simulink library "ammclib_bam_s32k14x"  (Simulink 9.0)
settings: Solver=ode45  StartTime=0.0  StopTime=10.0  RelTol=1e-3
undefined symbols (not defined in the file): f16A1, f16A2, f16B0, f16B1, f16B2, f16C1, f16CC1, f16CC1sc, f16CC1sc_D, f16CC1sc_Q, f16CC1scD, f16CC1scQ, f16CC2, f16CC2sc, f16CC2sc_D, f16CC2sc_Q, f16CC2scD, f16CC2scQ, f16DerivGain, f16EGain, f16FiltCoef, f16HystOff, f16HystOn, f16IGain, f16IntegGain, f16IntegGainFW, f16IntegGainQ, f16Kd, f16Kq, f16Limit, f16LowerLim, f16LowerLimit_D, f16LowerLimit_Q, f16ModIndex, f16OutValOff, f16OutValOn, f16PropGain, f16PropGainFW, f16PropGainQ, f16RampDown, f16RampUp, f16UGain, f16UpperLim, f16UpperLimit, f16UpperLimit_D, f16UpperLimit_Q, f16WIGain, f32A1, f32A2, f32B0, f32B1, f32B2, f32C1, f32CC1, f32CC1sc, f32CC1sc_D, f32CC1sc_Q, f32CC1scD, f32CC1scQ, f32CC2 ... (+122)
(part 2 of 11)

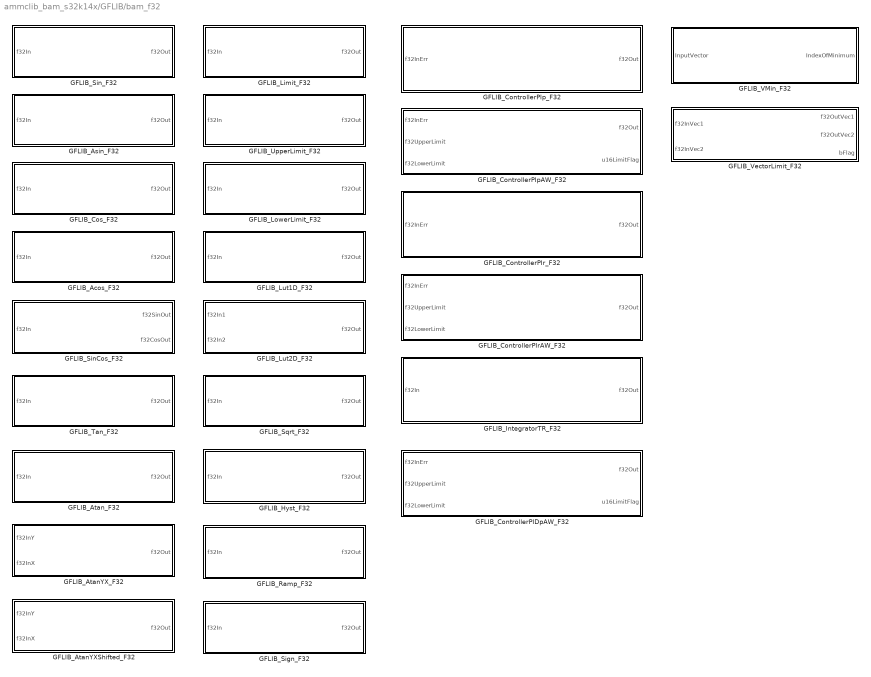
== system ammclib_bam_s32k14x/GFLIB/bam_f32 ==
  GFLIB_Acos_F32 : Subsystem  mask(GFLIB_Acos_F32){}
      mask help: Bit accurate model of GFLIB_Acos function, which computes the acos(fltIn) using the 4th order Taylor polynomial approximation.
      mask init:
      | pos = get_param(gcb, 'Position');width = pos(3) - pos(1); height = pos(4) - pos(2);tX=width/2;tY=height*0.9;
      mask Help: web(fullfile(mbd_s32k_mc_block_help('s32k14x'), 'S32K14XMCLUG.pdf'), '-browser')
      mask Display: color('black');port_label('input',1,'f32In');port_label('output',1,'f32Out');color('black');disp('GFLIB_Acos_F32');color('blue');text(tX,tY, 'BAM', 'horizontalAlignment', 'center');
  GFLIB_Asin_F32 : Subsystem  mask(GFLIB_Asin_F32){}
      mask help: Bit accurate model of GFLIB_Asin function, which computes the asin(f32In) using the 4th order Taylor polynomial approximation.
      mask init:
      | pos = get_param(gcb, 'Position');width = pos(3) - pos(1); height = pos(4) - pos(2);tX=width/2;tY=height*0.9;
      mask Help: web(fullfile(mbd_s32k_mc_block_help('s32k14x'), 'S32K14XMCLUG.pdf'), '-browser')
      mask Display: color('black');port_label('input',1,'f32In');port_label('output',1,'f32Out');color('black');disp('GFLIB_Asin_F32');color('blue');text(tX,tY, 'BAM', 'horizontalAlignment', 'center');
  GFLIB_AtanYXShifted_F32 : Subsystem  mask(GFLIB_AtanYXShifted_F32){Ky=Ky, Kx=Kx, Ny=Ny, Nx=Nx, ThetaAdj=ThetaAdj}
      mask help: Bit accurate model of GFLIB_AtanYXShifted function.
      mask init:
      | pos = get_param(gcb, 'Position');width = pos(3) - pos(1); height = pos(4) - pos(2);tX=width/2;tY=height*0.9;
      mask Help: web(fullfile(mbd_s32k_mc_block_help('s32k14x'), 'S32K14XMCLUG.pdf'), '-browser')
      mask Display: color('black');port_label('input',1,'f32InY');port_label('input',2,'f32InX');port_label('output',1,'f32Out');color('black');disp('GFLIB_AtanYXShifted_F32');color('blue');text(tX,tY, 'BAM', 'horizontalAlignment', 'center');
  GFLIB_AtanYX_F32 : Subsystem  mask(GFLIB_AtanYX_F32){}
      mask help: Bit accurate model of GFLIB_AtanYX function.
      mask init:
      | pos = get_param(gcb, 'Position');width = pos(3) - pos(1); height = pos(4) - pos(2);tX=width/2;tY=height*0.9;
      mask Help: web(fullfile(mbd_s32k_mc_block_help('s32k14x'), 'S32K14XMCLUG.pdf'), '-browser')
      mask Display: color('black');port_label('input',1,'f32InY');port_label('input',2,'f32InX');port_label('output',1,'f32Out');color('black');disp('GFLIB_AtanYX_F32');color('blue');text(tX,tY, 'BAM', 'horizontalAlignment', 'center');
  GFLIB_Atan_F32 : Subsystem  mask(GFLIB_Atan_F32){}
      mask help: Bit accurate model of GFLIB_Atan function, which computes the arctan(f32In) function.
      mask init:
      | pos = get_param(gcb, 'Position');width = pos(3) - pos(1); height = pos(4) - pos(2);tX=width/2;tY=height*0.9;
      mask Help: web(fullfile(mbd_s32k_mc_block_help('s32k14x'), 'S32K14XMCLUG.pdf'), '-browser')
      mask Display: color('black');port_label('input',1,'f32In');port_label('output',1,'f32Out');color('black');disp('GFLIB_Atan_F32');color('blue');text(tX,tY, 'BAM', 'horizontalAlignment', 'center');
  GFLIB_ControllerPIDpAW_F32 : Subsystem  mask(GFLIB_ControllerPIDpAW_F32){f32PropGain=f32PropGain, s16PropGainShift=s16PropGainShift, f32IntegGain=f32IntegGain, s16IntegGainShift=s16IntegGainShift, f32DerivGain=f32DerivGain, s16DerivGainShift=s16DerivGainShift, f32FiltCoef=f32FiltCoef}
      mask help: Bit accurate model of parallel form PID controller. All parameters as well as input and output are 32-bit integers except for s16xxxGainShift parameters which are 16-bit signed integers.
      mask init:
      | pos = get_param(gcb, 'Position');width = pos(3) - pos(1); height = pos(4) - pos(2);tX=width/2;tY=height*0.9;
      mask Help: web(fullfile(mbd_s32k_mc_block_help('s32k14x'), 'S32K14XMCLUG.pdf'), '-browser')
      mask Display: color('black');port_label('input',1,'f32InErr');port_label('input',2,'f32UpperLimit');port_label('input',3,'f32LowerLimit');port_label('output',1,'f32Out');port_label('output',2,'u16LimitFlag');color('black');disp('GFLIB_ControllerPIDpAW_F32');color('blue');text(tX,tY, 'BAM', 'horizontalAlignment', 'center');
  GFLIB_ControllerPIpAW_F32 : Subsystem  mask(GFLIB_ControllerPIpAW_F32){f32PropGain=f32PropGain, s16PropGainShift=s16PropGainShift, f32IntegGain=f32IntegGain, s16IntegGainShift=s16IntegGainShift}
      mask help: Bit accurate model of parallel form PI controller with anti-windup. All parameters as well as input and output are 32-bit integers except for u16NShift parameter which is 16-bit unsigned integer.
      mask init:
      | pos = get_param(gcb, 'Position');width = pos(3) - pos(1); height = pos(4) - pos(2);tX=width/2;tY=height*0.9;
      mask Help: web(fullfile(mbd_s32k_mc_block_help('s32k14x'), 'S32K14XMCLUG.pdf'), '-browser')
      mask Display: color('black');port_label('input',1,'f32InErr');port_label('input',2,'f32UpperLimit');port_label('input',3,'f32LowerLimit');port_label('output',1,'f32Out');port_label('output',2,'u16LimitFlag');color('black');disp('GFLIB_ControllerPIpAW_F32');color('blue');text(tX,tY, 'BAM', 'horizontalAlignment', 'center');
  GFLIB_ControllerPIp_F32 : Subsystem  mask(GFLIB_ControllerPIp_F32){f32PropGain=f32PropGain, s16PropGainShift=s16PropGainShift, f32IntegGain=f32IntegGain, s16IntegGainShift=s16IntegGainShift}
      mask help: Bit accurate model of parallel form PI controller. All parameters as well as input and output are 32-bit integers except for u16NShift parameter which is 16-bit unsigned integer.
      mask init:
      | pos = get_param(gcb, 'Position');width = pos(3) - pos(1); height = pos(4) - pos(2);tX=width/2;tY=height*0.9;
      mask Help: web(fullfile(mbd_s32k_mc_block_help('s32k14x'), 'S32K14XMCLUG.pdf'), '-browser')
      mask Display:
      | color('black');
      | port_label('input',1,'f32InErr');
      | port_label('output',1,'f32Out');
      | color('black');
      | disp('GFLIB_ControllerPIp_F32');
      | color('blue');
      | text(tX,tY, 'BAM', 'horizontalAlignment', 'center');
  GFLIB_ControllerPIrAW_F32 : Subsystem  mask(GFLIB_ControllerPIrAW_F32){f32CC1=f32CC1, f32CC2=f32CC2, u16NShift=u16NShift}
      mask help: Bit accurate model of reccurent form PI controller with anti-windup. All parameters as well as input and output are 32-bit integers except for u16NShift parameter which is 16-bit unsigned integer.
      mask init:
      | pos = get_param(gcb, 'Position');width = pos(3) - pos(1); height = pos(4) - pos(2);tX=width/2;tY=height*0.9;
      mask Help: web(fullfile(mbd_s32k_mc_block_help('s32k14x'), 'S32K14XMCLUG.pdf'), '-browser')
      mask Display: color('black');port_label('input',1,'f32InErr');port_label('input',2,'f32UpperLimit');port_label('input',3,'f32LowerLimit');port_label('output',1,'f32Out');color('black');disp('GFLIB_ControllerPIrAW_F32');color('blue');text(tX,tY, 'BAM', 'horizontalAlignment', 'center');
  GFLIB_ControllerPIr_F32 : Subsystem  mask(GFLIB_ControllerPIr_F32){f32CC1=f32CC1, f32CC2=f32CC2, u16NShift=u16NShift}
      mask help: Bit accurate model of reccurent form PI controller. All parameters as well as input and output are 32-bit integers except for u16NShift parameter which is 16-bit unsigned integer.
      mask init:
      | pos = get_param(gcb, 'Position');width = pos(3) - pos(1); height = pos(4) - pos(2);tX=width/2;tY=height*0.9;
      mask Help: web(fullfile(mbd_s32k_mc_block_help('s32k14x'), 'S32K14XMCLUG.pdf'), '-browser')
      mask Display:
      | color('black');
      | port_label('input',1,'f32InErr');
      | port_label('output',1,'f32Out');
      | color('black');
      | disp('GFLIB_ControllerPIr_F32');
      | color('blue');
      | text(tX,tY, 'BAM', 'horizontalAlignment', 'center');
  GFLIB_Cos_F32 : Subsystem  mask(GFLIB_Cos_F32){}
      mask help: Bit accurate model of GFLIB_Cos function, which computes the cos(f32In) using the 9th order Taylor polynomial approximation.
      mask init:
      | pos = get_param(gcb, 'Position');width = pos(3) - pos(1); height = pos(4) - pos(2);tX=width/2;tY=height*0.9;
      mask Help: web(fullfile(mbd_s32k_mc_block_help('s32k14x'), 'S32K14XMCLUG.pdf'), '-browser')
      mask Display: color('black');port_label('input',1,'f32In');port_label('output',1,'f32Out');color('black');disp('GFLIB_Cos_F32');color('blue');text(tX,tY, 'BAM', 'horizontalAlignment', 'center');
  GFLIB_Hyst_F32 : Subsystem  mask(GFLIB_Hyst_F32){f32HystOn=f32HystOn, f32HystOff=f32HystOff, f32OutValOn=f32OutValOn, f32OutValOff=f32OutValOff}
      mask help: Bit accurate model of hysteresis function. All parameters as well as input and output are 32-bit integers.
      mask init:
      | pos = get_param(gcb, 'Position');width = pos(3) - pos(1); height = pos(4) - pos(2);tX=width/2;tY=height*0.9;
      mask Help: web(fullfile(mbd_s32k_mc_block_help('s32k14x'), 'S32K14XMCLUG.pdf'), '-browser')
      mask Display: color('black');port_label('input',1,'f32In');port_label('output',1,'f32Out');color('black');disp('GFLIB_Hyst_F32');color('blue');text(tX,tY, 'BAM', 'horizontalAlignment', 'center');
  GFLIB_IntegratorTR_F32 : Subsystem  mask(GFLIB_IntegratorTR_F32){f32C1=f32C1, u16NShift=u16NShift}
      mask help: Bit accurate model of discrete trapezoidal integrator. All parameters as well as input and output are full float range.
      mask init:
      | pos = get_param(gcb, 'Position');width = pos(3) - pos(1); height = pos(4) - pos(2);tX=width/2;tY=height*0.9;
      mask Help: web(fullfile(mbd_s32k_mc_block_help('s32k14x'), 'S32K14XMCLUG.pdf'), '-browser')
      mask Display:
      | color('black');
      | port_label('input',1,'f32In');
      | port_label('output',1,'f32Out');
      | color('black');
      | disp('GFLIB_IntegratorTR_F32');
      | color('blue');
      | text(tX,tY, 'BAM', 'horizontalAlignment', 'center');
  GFLIB_Limit_F32 : Subsystem  mask(GFLIB_Limit){f32UpperLimit=f32UpperLimit, f32LowerLim=f32LowerLim}
      mask help: Bit accurate model of the GFLIB_Limit function.
      mask init:
      | pos = get_param(gcb, 'Position');width = pos(3) - pos(1); height = pos(4) - pos(2);tX=width/2;tY=height*0.9;
      mask Help: web(fullfile(mbd_s32k_mc_block_help('s32k14x'), 'S32K14XMCLUG.pdf'), '-browser')
      mask Display: color('black');port_label('input',1,'f32In');port_label('output',1,'f32Out');color('black');disp('GFLIB_Limit_F32');color('blue');text(tX,tY, 'BAM', 'horizontalAlignment', 'center');
  GFLIB_LowerLimit_F32 : Subsystem  mask(GFLIB_LowerLimit_F32){f32LowerLim=f32LowerLim}
      mask help: Bit accurate model of GFLIB_LowerLimit function.
      mask init:
      | pos = get_param(gcb, 'Position');width = pos(3) - pos(1); height = pos(4) - pos(2);tX=width/2;tY=height*0.9;
      mask Help: web(fullfile(mbd_s32k_mc_block_help('s32k14x'), 'S32K14XMCLUG.pdf'), '-browser')
      mask Display: color('black');port_label('input',1,'f32In');port_label('output',1,'f32Out');color('black');disp('GFLIB_LowerLimit_F32');color('blue');text(tX,tY, 'BAM', 'horizontalAlignment', 'center');
  GFLIB_Lut1D_F32 : Subsystem  mask(GFLIB_Lut1D_F32){u32ShamOffset=u32ShamOffset, pf32Table=pf32Table, s32MidIdx=s32MidIdx}
      mask help: Bit accurate model of Lut1D function.
      mask init:
      | pos = get_param(gcb, 'Position');width = pos(3) - pos(1); height = pos(4) - pos(2);tX=width/2;tY=height*0.9;
      mask Help: web(fullfile(mbd_s32k_mc_block_help('s32k14x'), 'S32K14XMCLUG.pdf'), '-browser')
      mask Display: color('black');port_label('input',1,'f32In');port_label('output',1,'f32Out');color('black');disp('GFLIB_Lut1D_F32');color('blue');text(tX,tY, 'BAM', 'horizontalAlignment', 'center');
  GFLIB_Lut2D_F32 : Subsystem  mask(GFLIB_Lut2D_F32){u32ShamOffset1=u32ShamOffset1, u32ShamOffset2=u32ShamOffset2, pf32Table=pf32Table, s32MidIdx=s32MidIdx}
      mask help: Bit accurate model of Lut2D function.
      mask init:
      | pos = get_param(gcb, 'Position');width = pos(3) - pos(1); height = pos(4) - pos(2);tX=width/2;tY=height*0.9;
      mask Help: web(fullfile(mbd_s32k_mc_block_help('s32k14x'), 'S32K14XMCLUG.pdf'), '-browser')
      mask Display: color('black');port_label('input',1,'f32In1');port_label('input',2,'f32In2');port_label('output',1,'f32Out');color('black');disp('GFLIB_Lut2D_F32');color('blue');text(tX,tY, 'BAM', 'horizontalAlignment', 'center');
  GFLIB_Ramp_F32 : Subsystem  mask(GFLIB_Ramp){f32RampUp=f32RampUp, f32RampDown=f32RampDown}
      mask help: Bit accurate model of ramp function. All parameters as well as input and output are 32bit integers.
      mask init:
      | pos = get_param(gcb, 'Position');width = pos(3) - pos(1); height = pos(4) - pos(2);tX=width/2;tY=height*0.9;
      mask Help: web(fullfile(mbd_s32k_mc_block_help('s32k14x'), 'S32K14XMCLUG.pdf'), '-browser')
      mask Display: color('black');port_label('input',1,'f32In');port_label('output',1,'f32Out');color('black');disp('GFLIB_Ramp_F32');color('blue');text(tX,tY, 'BAM', 'horizontalAlignment', 'center');
  GFLIB_Sign_F32 : Subsystem  mask(GFLIB_Sign_F32){}
      mask help: Bit accurate model of GFLIB_Sign function.
      mask init:
      | pos = get_param(gcb, 'Position');width = pos(3) - pos(1); height = pos(4) - pos(2);tX=width/2;tY=height*0.9;
      mask Help: web(fullfile(mbd_s32k_mc_block_help('s32k14x'), 'S32K14XMCLUG.pdf'), '-browser')
      mask Display: color('black');port_label('input',1,'f32In');port_label('output',1,'f32Out');color('black');disp('GFLIB_Sign_F32');color('blue');text(tX,tY, 'BAM', 'horizontalAlignment', 'center');
  GFLIB_SinCos_F32 : Subsystem  mask(GFLIB_SinCos_F32){}
      mask help: Bit accurate model of GFLIB_SinCos function, which computes the sin(f32n) and cos(f32In) using the 9th order Taylor polynomial approximation.
      mask init:
      | pos = get_param(gcb, 'Position');width = pos(3) - pos(1); height = pos(4) - pos(2);tX=width/2;tY=height*0.9;
      mask Help: web(fullfile(mbd_s32k_mc_block_help('s32k14x'), 'S32K14XMCLUG.pdf'), '-browser')
      mask Display: color('black');port_label('input',1,'f32In');port_label('output',1,'f32SinOut');port_label('output',2,'f32CosOut');color('black');disp('GFLIB_SinCos_F32');color('blue');text(tX,tY, 'BAM', 'horizontalAlignment', 'center');
  GFLIB_Sin_F32 : Subsystem  mask(GFLIB_Sin_F32){}
      mask help: Bit accurate model of GFLIB_Sin function, which computes the sin(f32n) using the 9th order Taylor polynomial approximation.
      mask init:
      | pos = get_param(gcb, 'Position');width = pos(3) - pos(1); height = pos(4) - pos(2);tX=width/2;tY=height*0.9;
      mask Help: web(fullfile(mbd_s32k_mc_block_help('s32k14x'), 'S32K14XMCLUG.pdf'), '-browser')
      mask Display: color('black');port_label('input',1,'f32In');port_label('output',1,'f32Out');color('black');disp('GFLIB_Sin_F32');color('blue');text(tX,tY, 'BAM', 'horizontalAlignment', 'center');
  GFLIB_Sqrt_F32 : Subsystem  mask(GFLIB_Sqrt_F32){}
      mask help: Bit accurate model of GFLIB_Sqrt function, which computes the square root of input value.
      mask init:
      | pos = get_param(gcb, 'Position');width = pos(3) - pos(1); height = pos(4) - pos(2);tX=width/2;tY=height*0.9;
      mask Help: web(fullfile(mbd_s32k_mc_block_help('s32k14x'), 'S32K14XMCLUG.pdf'), '-browser')
      mask Display: color('black');port_label('input',1,'f32In');port_label('output',1,'f32Out');color('black');disp('GFLIB_Sqrt_F32');color('blue');text(tX,tY, 'BAM', 'horizontalAlignment', 'center');
  GFLIB_Tan_F32 : Subsystem  mask(GFLIB_Tan_F32){}
      mask help: Bit accurate model of GFLIB_Tan function, which computes the tan(f32In) function.
      mask init:
      | pos = get_param(gcb, 'Position');width = pos(3) - pos(1); height = pos(4) - pos(2);tX=width/2;tY=height*0.9;
      mask Help: web(fullfile(mbd_s32k_mc_block_help('s32k14x'), 'S32K14XMCLUG.pdf'), '-browser')
      mask Display: color('black');port_label('input',1,'f32In');port_label('output',1,'f32Out');color('black');disp('GFLIB_Tan_F32');color('blue');text(tX,tY, 'BAM', 'horizontalAlignment', 'center');
  GFLIB_UpperLimit_F32 : Subsystem  mask(GFLIB_UpperLimit_F32){f32UpperLim=f32UpperLim}
      mask help: Bit accurate model of GFLIB_UpperLimit function.
      mask init:
      | pos = get_param(gcb, 'Position');width = pos(3) - pos(1); height = pos(4) - pos(2);tX=width/2;tY=height*0.9;
      mask Help: web(fullfile(mbd_s32k_mc_block_help('s32k14x'), 'S32K14XMCLUG.pdf'), '-browser')
      mask Display: color('black');port_label('input',1,'f32In');port_label('output',1,'f32Out');color('black');disp('GFLIB_UpperLimit_F32');color('blue');text(tX,tY, 'BAM', 'horizontalAlignment', 'center');
  GFLIB_VMin_F32 : Subsystem  mask(GFLIB_VMin_F32){N=N}
      mask prompts: N "Vector length"
      mask help: Bit accurate model of GFLIB_VMin function, which finds the index of a vector minimum.
      mask init:
      | pos = get_param(gcb, 'Position');width = pos(3) - pos(1); height = pos(4) - pos(2);tX=width/2;tY=height*0.9;
      mask Help: web(fullfile(mbd_s32k_mc_block_help('s32k14x'), 'S32K14XMCLUG.pdf'), '-browser')
      mask Display: color('black');port_label('input',1,'InputVector');port_label('output',1,'IndexOfMinimum');color('black');disp('GFLIB_VMin_F32');color('blue');text(tX,tY, 'BAM', 'horizontalAlignment', 'center');
  GFLIB_VectorLimit_F32 : Subsystem  mask(GFLIB_VectorLimit){f32Limit=f32Limit}
      mask help: Bit accurate model of the GFLIB_VectorLimit function.
      mask init:
      | pos = get_param(gcb, 'Position');width = pos(3) - pos(1); height = pos(4) - pos(2);tX=width/2;tY=height*0.9;
      mask Help: web(fullfile(mbd_s32k_mc_block_help('s32k14x'), 'S32K14XMCLUG.pdf'), '-browser')
      mask Display: color('black');port_label('input',1,'f32InVec1');port_label('input',2,'f32InVec2');port_label('output',1,'f32OutVec1');port_label('output',2,'f32OutVec2');port_label('output',3,'bFlag');color('black');disp('GFLIB_VectorLimit_F32');color('blue');text(tX,tY, 'BAM', 'horizontalAlignment', 'center');

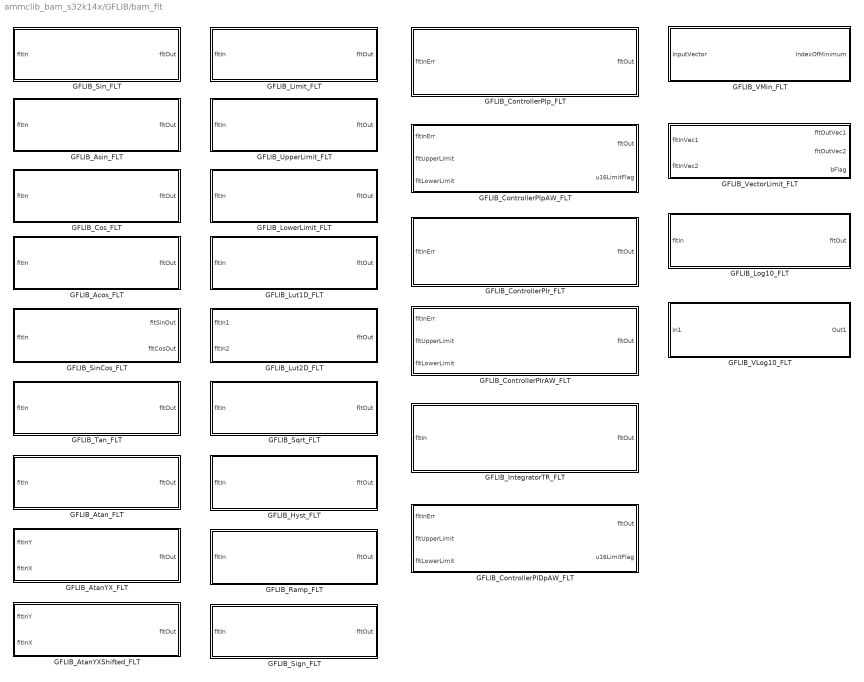
== system ammclib_bam_s32k14x/GFLIB/bam_flt ==
  GFLIB_Acos_FLT : Subsystem  mask(GFLIB_Acos_FLT){}
      mask help: Bit accurate model of GFLIB_Acos function, which computes the acos(fltIn) using the square based approximation.
      mask init:
      | pos = get_param(gcb, 'Position');width = pos(3) - pos(1); height = pos(4) - pos(2);tX=width/2;tY=height*0.9;
      mask Help: web(fullfile(mbd_s32k_mc_block_help('s32k14x'), 'S32K14XMCLUG.pdf'), '-browser')
      mask Display: color('black');port_label('input',1,'fltIn');port_label('output',1,'fltOut');color('black');disp('GFLIB_Acos_FLT');color('blue');text(tX,tY, 'BAM', 'horizontalAlignment', 'center');
  GFLIB_Asin_FLT : Subsystem  mask(GFLIB_Asin_FLT){}
      mask help: Bit accurate model of GFLIB_Asin function, which computes the asin(fltIn) using the square based approximation.
      mask init:
      | pos = get_param(gcb, 'Position');width = pos(3) - pos(1); height = pos(4) - pos(2);tX=width/2;tY=height*0.9;
      mask Help: web(fullfile(mbd_s32k_mc_block_help('s32k14x'), 'S32K14XMCLUG.pdf'), '-browser')
      mask Display: color('black');port_label('input',1,'fltIn');port_label('output',1,'fltOut');color('black');disp('GFLIB_Asin_FLT');color('blue');text(tX,tY, 'BAM', 'horizontalAlignment', 'center');
  GFLIB_AtanYXShifted_FLT : Subsystem  mask(GFLIB_AtanYXShifted_FLT){Ky=Ky, Kx=Kx, ThetaAdj=ThetaAdj}
      mask help: Bit accurate model of GFLIB_AtanYXShifted function.
      mask init:
      | pos = get_param(gcb, 'Position');width = pos(3) - pos(1); height = pos(4) - pos(2);tX=width/2;tY=height*0.9;
      mask Help: web(fullfile(mbd_s32k_mc_block_help('s32k14x'), 'S32K14XMCLUG.pdf'), '-browser')
      mask Display: color('black');port_label('input',1,'fltInY');port_label('input',2,'fltInX');port_label('output',1,'fltOut');color('black');disp('GFLIB_AtanYXShifted_FLT');color('blue');text(tX,tY, 'BAM', 'horizontalAlignment', 'center');
  GFLIB_AtanYX_FLT : Subsystem  mask(GFLIB_AtanYX_FLT){}
      mask help: Bit accurate model of GFLIB_AtanYX function.
      mask init:
      | pos = get_param(gcb, 'Position');width = pos(3) - pos(1); height = pos(4) - pos(2);tX=width/2;tY=height*0.9;
      mask Help: web(fullfile(mbd_s32k_mc_block_help('s32k14x'), 'S32K14XMCLUG.pdf'), '-browser')
      mask Display: color('black');port_label('input',1,'fltInY');port_label('input',2,'fltInX');port_label('output',1,'fltOut');color('black');disp('GFLIB_AtanYX_FLT');color('blue');text(tX,tY, 'BAM', 'horizontalAlignment', 'center');
  GFLIB_Atan_FLT : Subsystem  mask(GFLIB_Atan_FLT){}
      mask help: Bit accurate model of GFLIB_Atan function, which computes the arctan(fltIn) function.
      mask init:
      | pos = get_param(gcb, 'Position');width = pos(3) - pos(1); height = pos(4) - pos(2);tX=width/2;tY=height*0.9;
      mask Help: web(fullfile(mbd_s32k_mc_block_help('s32k14x'), 'S32K14XMCLUG.pdf'), '-browser')
      mask Display: color('black');port_label('input',1,'fltIn');port_label('output',1,'fltOut');color('black');disp('GFLIB_Atan_FLT');color('blue');text(tX,tY, 'BAM', 'horizontalAlignment', 'center');
  GFLIB_ControllerPIDpAW_FLT : Subsystem  mask(GFLIB_ControllerPIDpAW_FLT){fltPropGain=fltPropGain, fltIntegGain=fltIntegGain, fltDerivGain=fltDerivGain, fltFiltCoef=fltFiltCoef}
      mask help: Bit accurate model of parallel form PID controller. All parameters as well as input and output are single precison floating point numbers with exception of u16LimitFlag, which is 16-bit unsigned integer.
      mask init:
      | pos = get_param(gcb, 'Position');width = pos(3) - pos(1); height = pos(4) - pos(2);tX=width/2;tY=height*0.9;
      mask Help: web(fullfile(mbd_s32k_mc_block_help('s32k14x'), 'S32K14XMCLUG.pdf'), '-browser')
      mask Display: color('black');port_label('input',1,'fltInErr');port_label('input',2,'fltUpperLimit');port_label('input',3,'fltLowerLimit');port_label('output',1,'fltOut');port_label('output',2,'u16LimitFlag');color('black');disp('GFLIB_ControllerPIDpAW_FLT');color('blue');text(tX,tY, 'BAM', 'horizontalAlignment', 'center');
  GFLIB_ControllerPIpAW_FLT : Subsystem  mask(GFLIB_ControllerPIpAW_FLT){fltPropGain=fltPropGain, fltIntegGain=fltIntegGain}
      mask help: Bit accurate model of parallel form PI controller with anti-windup. All parameters as well as input and output are single precison floating point numbers with exception of u16LimitFlag, which is 16-bit unsigned integer.
      mask init:
      | pos = get_param(gcb, 'Position');width = pos(3) - pos(1); height = pos(4) - pos(2);tX=width/2;tY=height*0.9;
      mask Help: web(fullfile(mbd_s32k_mc_block_help('s32k14x'), 'S32K14XMCLUG.pdf'), '-browser')
      mask Display: color('black');port_label('input',1,'fltInErr');port_label('input',2,'fltUpperLimit');port_label('input',3,'fltLowerLimit');port_label('output',1,'fltOut');port_label('output',2,'u16LimitFlag');color('black');disp('GFLIB_ControllerPIpAW_FLT');color('blue');text(tX,tY, 'BAM', 'horizontalAlignment', 'center');
  GFLIB_ControllerPIp_FLT : Subsystem  mask(GFLIB_ControllerPIp_FLT){fltPropGain=fltPropGain, fltIntegGain=fltIntegGain}
      mask help: Bit accurate model of parallel form PI controller. All parameters as well as input and output are single precison floating point numbers with exception of u16LimitFlag, which is 16-bit unsigned integer.
      mask init:
      | pos = get_param(gcb, 'Position');width = pos(3) - pos(1); height = pos(4) - pos(2);tX=width/2;tY=height*0.9;
      mask Help: web(fullfile(mbd_s32k_mc_block_help('s32k14x'), 'S32K14XMCLUG.pdf'), '-browser')
      mask Display:
      | color('black');
      | port_label('input',1,'fltInErr');
      | port_label('output',1,'fltOut');
      | color('black');
      | disp('GFLIB_ControllerPIp_FLT');
      | color('blue');
      | text(tX,tY, 'BAM', 'horizontalAlignment', 'center');
  GFLIB_ControllerPIrAW_FLT : Subsystem  mask(GFLIB_ControllerPIrAW_FLT){fltCC1=fltCC1, fltCC2=fltCC2}
      mask help: Bit accurate model of reccurent form PI controller with anti-windup. All parameters as well as input and output are single precison floating point numbers.
      mask init:
      | pos = get_param(gcb, 'Position');width = pos(3) - pos(1); height = pos(4) - pos(2);tX=width/2;tY=height*0.9;
      mask Help: web(fullfile(mbd_s32k_mc_block_help('s32k14x'), 'S32K14XMCLUG.pdf'), '-browser')
      mask Display: color('black');port_label('input',1,'fltInErr');port_label('input',2,'fltUpperLimit');port_label('input',3,'fltLowerLimit');port_label('output',1,'fltOut');color('black');disp('GFLIB_ControllerPIrAW_FLT');color('blue');text(tX,tY, 'BAM', 'horizontalAlignment', 'center');
  GFLIB_ControllerPIr_FLT : Subsystem  mask(GFLIB_ControllerPIr_FLT){fltCC1=fltCC1, fltCC2=fltCC2}
      mask help: Bit accurate model of reccurent form PI controller. All parameters as well as input and output are single precison floating point numbers.
      mask init:
      | pos = get_param(gcb, 'Position');width = pos(3) - pos(1); height = pos(4) - pos(2);tX=width/2;tY=height*0.9;
      mask Help: web(fullfile(mbd_s32k_mc_block_help('s32k14x'), 'S32K14XMCLUG.pdf'), '-browser')
      mask Display:
      | color('black');
      | port_label('input',1,'fltInErr');
      | port_label('output',1,'fltOut');
      | color('black');
      | disp('GFLIB_ControllerPIr_FLT');
      | color('blue');
      | text(tX,tY, 'BAM', 'horizontalAlignment', 'center');
  GFLIB_Cos_FLT : Subsystem  mask(GFLIB_Cos_FLT){}
      mask help: Bit accurate model of GFLIB_Cos function, which computes the cos(fltIn) using the floating point optimized approximation.
      mask init:
      | pos = get_param(gcb, 'Position');width = pos(3) - pos(1); height = pos(4) - pos(2);tX=width/2;tY=height*0.9;
      mask Help: web(fullfile(mbd_s32k_mc_block_help('s32k14x'), 'S32K14XMCLUG.pdf'), '-browser')
      mask Display: color('black');port_label('input',1,'fltIn');port_label('output',1,'fltOut');color('black');disp('GFLIB_Cos_FLT');color('blue');text(tX,tY, 'BAM', 'horizontalAlignment', 'center');
  GFLIB_Hyst_FLT : Subsystem  mask(GFLIB_Hyst_FLT){fltHystOn=fltHystOn, fltHystOff=fltHystOff, fltOutValOn=fltOutValOn, fltOutValOff=fltOutValOff}
      mask help: Bit accurate model of hysteresis function. All parameters as well as input and output are in a full float range.
      mask init:
      | pos = get_param(gcb, 'Position');width = pos(3) - pos(1); height = pos(4) - pos(2);tX=width/2;tY=height*0.9;
      mask Help: web(fullfile(mbd_s32k_mc_block_help('s32k14x'), 'S32K14XMCLUG.pdf'), '-browser')
      mask Display: color('black');port_label('input',1,'fltIn');port_label('output',1,'fltOut');color('black');disp('GFLIB_Hyst_FLT');color('blue');text(tX,tY, 'BAM', 'horizontalAlignment', 'center');
  GFLIB_IntegratorTR_FLT : Subsystem  mask(GFLIB_IntegratorTR_FLT){fltC1=fltC1}
      mask help: Bit accurate model of discrete trapezoidal integrator. All parameters as well as input and output are full float range.
      mask init:
      | pos = get_param(gcb, 'Position');width = pos(3) - pos(1); height = pos(4) - pos(2);tX=width/2;tY=height*0.9;
      mask Help: web(fullfile(mbd_s32k_mc_block_help('s32k14x'), 'S32K14XMCLUG.pdf'), '-browser')
      mask Display:
      | color('black');
      | port_label('input',1,'fltIn');
      | port_label('output',1,'fltOut');
      | color('black');
      | disp('GFLIB_IntegratorTR_FLT');
      | color('blue');
      | text(tX,tY, 'BAM', 'horizontalAlignment', 'center');
  GFLIB_Limit_FLT : Subsystem  mask(GFLIB_Limit){fltUpperLimit=fltUpperLimit, fltLowerLim=fltLowerLim}
      mask help: Bit accurate model of the GFLIB_Limit function.
      mask init:
      | pos = get_param(gcb, 'Position');width = pos(3) - pos(1); height = pos(4) - pos(2);tX=width/2;tY=height*0.9;
      mask Help: web(fullfile(mbd_s32k_mc_block_help('s32k14x'), 'S32K14XMCLUG.pdf'), '-browser')
      mask Display: color('black');port_label('input',1,'fltIn');port_label('output',1,'fltOut');color('black');disp('GFLIB_Limit_FLT');color('blue');text(tX,tY, 'BAM', 'horizontalAlignment', 'center');
  GFLIB_Log10_FLT : Subsystem  mask(GFLIB_Log10_FLT){}
      mask help: Bit accurate model of GFLIB_Log10 function, which computes fast base-10 logarithm.
      mask init:
      | pos = get_param(gcb, 'Position');width = pos(3) - pos(1); height = pos(4) - pos(2);tX=width/2;tY=height*0.9;
      mask Help: web(fullfile(mbd_s32k_mc_block_help('s32k14x'), 'S32K14XMCLUG.pdf'), '-browser')
      mask Display: color('black');port_label('input',1,'fltIn');port_label('output',1,'fltOut');color('black');disp('GFLIB_Log10_FLT');color('blue');text(tX,tY, 'BAM', 'horizontalAlignment', 'center');
  GFLIB_LowerLimit_FLT : Subsystem  mask(GFLIB_LowerLimit_FLT){fltLowerLim=fltLowerLim}
      mask help: Bit accurate model of GFLIB_LowerLimit function.
      mask init:
      | pos = get_param(gcb, 'Position');width = pos(3) - pos(1); height = pos(4) - pos(2);tX=width/2;tY=height*0.9;
      mask Help: web(fullfile(mbd_s32k_mc_block_help('s32k14x'), 'S32K14XMCLUG.pdf'), '-browser')
      mask Display: color('black');port_label('input',1,'fltIn');port_label('output',1,'fltOut');color('black');disp('GFLIB_LowerLimit_FLT');color('blue');text(tX,tY, 'BAM', 'horizontalAlignment', 'center');
  GFLIB_Lut1D_FLT : Subsystem  mask(GFLIB_Lut1D_FLT){u32ShamOffset=u32ShamOffset, pfltTable=pfltTable, s32MidIdx=s32MidIdx}
      mask help: Bit accurate model of Lut1D function.
      mask init:
      | pos = get_param(gcb, 'Position');width = pos(3) - pos(1); height = pos(4) - pos(2);tX=width/2;tY=height*0.9;
      mask Help: web(fullfile(mbd_s32k_mc_block_help('s32k14x'), 'S32K14XMCLUG.pdf'), '-browser')
      mask Display: color('black');port_label('input',1,'fltIn');port_label('output',1,'fltOut');color('black');disp('GFLIB_Lut1D_FLT');color('blue');text(tX,tY, 'BAM', 'horizontalAlignment', 'center');
  GFLIB_Lut2D_FLT : Subsystem  mask(GFLIB_Lut2D_FLT){u32ShamOffset1=u32ShamOffset1, u32ShamOffset2=u32ShamOffset2, pfltTable=pfltTable, s32MidIdx=s32MidIdx}
      mask help: Bit accurate model of Lut2D function.
      mask init:
      | pos = get_param(gcb, 'Position');width = pos(3) - pos(1); height = pos(4) - pos(2);tX=width/2;tY=height*0.9;
      mask Help: web(fullfile(mbd_s32k_mc_block_help('s32k14x'), 'S32K14XMCLUG.pdf'), '-browser')
      mask Display: color('black');port_label('input',1,'fltIn1');port_label('input',2,'fltIn2');port_label('output',1,'fltOut');color('black');disp('GFLIB_Lut2D_FLT');color('blue');text(tX,tY, 'BAM', 'horizontalAlignment', 'center');
  GFLIB_Ramp_FLT : Subsystem  mask(GFLIB_Ramp){fltRampUp=fltRampUp, fltRampDown=fltRampDown}
      mask help: Bit accurate model of ramp function. All parameters as well as input and output are in single precision floating data format.
      mask init:
      | pos = get_param(gcb, 'Position');width = pos(3) - pos(1); height = pos(4) - pos(2);tX=width/2;tY=height*0.9;
      mask Help: web(fullfile(mbd_s32k_mc_block_help('s32k14x'), 'S32K14XMCLUG.pdf'), '-browser')
      mask Display: color('black');port_label('input',1,'fltIn');port_label('output',1,'fltOut');color('black');disp('GFLIB_Ramp_FLT');color('blue');text(tX,tY, 'BAM', 'horizontalAlignment', 'center');
  GFLIB_Sign_FLT : Subsystem  mask(GFLIB_Sign_FLT){}
      mask help: Bit accurate model of the GFLIB_Sign function.
      mask init:
      | pos = get_param(gcb, 'Position');width = pos(3) - pos(1); height = pos(4) - pos(2);tX=width/2;tY=height*0.9;
      mask Help: web(fullfile(mbd_s32k_mc_block_help('s32k14x'), 'S32K14XMCLUG.pdf'), '-browser')
      mask Display: color('black');port_label('input',1,'fltIn');port_label('output',1,'fltOut');color('black');disp('GFLIB_Sign_FLT');color('blue');text(tX,tY, 'BAM', 'horizontalAlignment', 'center');
  GFLIB_SinCos_FLT : Subsystem  mask(GFLIB_SinCos_FLT){}
      mask help: Bit accurate model of GFLIB_SinCos function, which computes the sin(fltIn) and cos(fltIn) using the floating point optimized approximation.
      mask init:
      | pos = get_param(gcb, 'Position');width = pos(3) - pos(1); height = pos(4) - pos(2);tX=width/2;tY=height*0.9;
      mask Help: web(fullfile(mbd_s32k_mc_block_help('s32k14x'), 'S32K14XMCLUG.pdf'), '-browser')
      mask Display: color('black');port_label('input',1,'fltIn');port_label('output',1,'fltSinOut');port_label('output',2,'fltCosOut');color('black');disp('GFLIB_SinCos_FLT');color('blue');text(tX,tY, 'BAM', 'horizontalAlignment', 'center');
  GFLIB_Sin_FLT : Subsystem  mask(GFLIB_Sin_FLT){}
      mask help: Bit accurate model of GFLIB_Sin function, which computes the sin(fltIn) using the floating point optimized approximation.
      mask init:
      | pos = get_param(gcb, 'Position');width = pos(3) - pos(1); height = pos(4) - pos(2);tX=width/2;tY=height*0.9;
      mask Help: web(fullfile(mbd_s32k_mc_block_help('s32k14x'), 'S32K14XMCLUG.pdf'), '-browser')
      mask Display: color('black');port_label('input',1,'fltIn');port_label('output',1,'fltOut');color('black');disp('GFLIB_Sin_FLT');color('blue');text(tX,tY, 'BAM', 'horizontalAlignment', 'center');
  GFLIB_Sqrt_FLT : Subsystem  mask(GFLIB_Sqrt_FLT){}
      mask help: Bit accurate model of GFLIB_Sqrt function, which computes the square root of input value.
      mask init:
      | pos = get_param(gcb, 'Position');width = pos(3) - pos(1); height = pos(4) - pos(2);tX=width/2;tY=height*0.9;
      mask Help: web(fullfile(mbd_s32k_mc_block_help('s32k14x'), 'S32K14XMCLUG.pdf'), '-browser')
      mask Display: color('black');port_label('input',1,'fltIn');port_label('output',1,'fltOut');color('black');disp('GFLIB_Sqrt_FLT');color('blue');text(tX,tY, 'BAM', 'horizontalAlignment', 'center');
  GFLIB_Tan_FLT : Subsystem  mask(GFLIB_Tan_FLT){}
      mask help: Bit accurate model of GFLIB_Tan function, which computes the tan(fltIn) function.
      mask init:
      | pos = get_param(gcb, 'Position');width = pos(3) - pos(1); height = pos(4) - pos(2);tX=width/2;tY=height*0.9;
      mask Help: web(fullfile(mbd_s32k_mc_block_help('s32k14x'), 'S32K14XMCLUG.pdf'), '-browser')
      mask Display: color('black');port_label('input',1,'fltIn');port_label('output',1,'fltOut');color('black');disp('GFLIB_Tan_FLT');color('blue');text(tX,tY, 'BAM', 'horizontalAlignment', 'center');
  GFLIB_UpperLimit_FLT : Subsystem  mask(GFLIB_UpperLimit_FLT){fltUpperLim=fltUpperLim}
      mask help: Bit accurate model of GFLIB_UpperLimit function.
      mask init:
      | pos = get_param(gcb, 'Position');width = pos(3) - pos(1); height = pos(4) - pos(2);tX=width/2;tY=height*0.9;
      mask Help: web(fullfile(mbd_s32k_mc_block_help('s32k14x'), 'S32K14XMCLUG.pdf'), '-browser')
      mask Display: color('black');port_label('input',1,'fltIn');port_label('output',1,'fltOut');color('black');disp('GFLIB_UpperLimit_FLT');color('blue');text(tX,tY, 'BAM', 'horizontalAlignment', 'center');
  GFLIB_VLog10_FLT : Subsystem  mask(GFLIB_VLog10_FLT){N=32}
      mask prompts: N "Vector length"
      mask help:
      | Bit accurate model of GFLIB_VLog10 function, which computes fast base-10 logarithm of a vector.
      |
      | Note: The vector length parameter N must be <= 4096.
      mask Help: web(fullfile(mbd_s32k_mc_block_help('s32k14x'), 'S32K14XMCLUG.pdf'), '-browser')
      mask Display:
      | color('black');
      | port_label('input',1,'fltIn');
      | port_label('output',1,'fltOut');
      | color('black');
      | disp('GFLIB_VLog10_FLT');
  GFLIB_VMin_FLT : Subsystem  mask(GFLIB_VMin_FLT){N=N}
      mask prompts: N "Vector length"
      mask help: Bit accurate model of GFLIB_VMin function, which finds the index of a vector minimum.
      mask init:
      | pos = get_param(gcb, 'Position');width = pos(3) - pos(1); height = pos(4) - pos(2);tX=width/2;tY=height*0.9;
      mask Help: web(fullfile(mbd_s32k_mc_block_help('s32k14x'), 'S32K14XMCLUG.pdf'), '-browser')
      mask Display: color('black');port_label('input',1,'InputVector');port_label('output',1,'IndexOfMinimum');color('black');disp('GFLIB_VMin_FLT');color('blue');text(tX,tY, 'BAM', 'horizontalAlignment', 'center');
  GFLIB_VectorLimit_FLT : Subsystem  mask(GFLIB_VectorLimit){fltLimit=fltLimit}
      mask help: Bit accurate model of the GFLIB_VectorLimit function.
      mask init:
      | pos = get_param(gcb, 'Position');width = pos(3) - pos(1); height = pos(4) - pos(2);tX=width/2;tY=height*0.9;
      mask Help: web(fullfile(mbd_s32k_mc_block_help('s32k14x'), 'S32K14XMCLUG.pdf'), '-browser')
      mask Display: color('black');port_label('input',1,'fltInVec1');port_label('input',2,'fltInVec2');port_label('output',1,'fltOutVec1');port_label('output',2,'fltOutVec2');port_label('output',3,'bFlag');color('black');disp('GFLIB_VectorLimit_FLT');color('blue');text(tX,tY, 'BAM', 'horizontalAlignment', 'center');

== system ammclib_bam_s32k14x/GMCLIB/bam_f16 ==
  GMCLIB_ClarkInv_F16 : Subsystem  mask(GMCLIB_ClarkInv_F16){}
      mask help: Bit accurate model of inverse Clarke transformation 2ph -> 3ph
      mask init:
      | pos = get_param(gcb, 'Position');width = pos(3) - pos(1); height = pos(4) - pos(2);tX=width/2;tY=height*0.9;
      mask Help: web(fullfile(mbd_s32k_mc_block_help('s32k14x'), 'S32K14XMCLUG.pdf'), '-browser')
      mask Display: color('black');port_label('input',1,'f16Alpha');port_label('input',2,'f16Beta');port_label('output',1,'f16A');port_label('output',2,'f16B');port_label('output',3,'f16C');color('black');disp('GMCLIB_ClarkInv_F16');color('blue');text(tX,tY, 'BAM', 'horizontalAlignment', 'center');
  GMCLIB_Clark_F16 : Subsystem  mask(GMCLIB_Clark_F16){}
      mask help: Bit accurate model of Clarke transformation 3ph -> 2ph.
      mask init:
      | pos = get_param(gcb, 'Position');width = pos(3) - pos(1); height = pos(4) - pos(2);tX=width/2;tY=height*0.9;
      mask Help: web(fullfile(mbd_s32k_mc_block_help('s32k14x'), 'S32K14XMCLUG.pdf'), '-browser')
      mask Display: color('black');port_label('input',1,'f16A');port_label('input',2,'f16B');port_label('input',3,'f16C');port_label('output',1,'f16Alpha');port_label('output',2,'f16Beta');color('black');disp('GMCLIB_Clark_F16');color('blue');text(tX,tY, 'BAM', 'horizontalAlignment', 'center');
  GMCLIB_DecouplingPMSM_F16 : Subsystem  mask(GMCLIB_DecouplingPMSM_F16){f16Kd=f16Kd, s16KdShift=s16KdShift, f16Kq=f16Kq, s16KqShift=s16KqShift}
      mask help: Bit accurate model of decoupling for PMSM model.
      mask init:
      | pos = get_param(gcb, 'Position');width = pos(3) - pos(1); height = pos(4) - pos(2);tX=width/2;tY=height*0.9;
      mask Help: web(fullfile(mbd_s32k_mc_block_help('s32k14x'), 'S32K14XMCLUG.pdf'), '-browser')
      mask Display: color('black');port_label('input',1,'f16Ud');port_label('input',2,'f16Uq');port_label('input',3,'f16Id');port_label('input',4,'f16Iq');port_label('input',5,'f16AngVel');port_label('output',1,'f16UdDec');port_label('output',2,'f16UqDec');color('black');disp('GMCLIB_DecouplingPMSM_F16');color('blue');text(tX,tY, 'BAM', 'horizontalAlignment', 'center');
  GMCLIB_ElimDcBusRip_F16 : Subsystem  mask(GMCLIB_ElimDcBusRip_F16){f16ModIndex=f16ModIndex}
      mask help: Bit accurate model of DC Bus voltage ripple elimination function.
      mask init:
      | pos = get_param(gcb, 'Position');width = pos(3) - pos(1); height = pos(4) - pos(2);tX=width/2;tY=height*0.9;
      mask Help: web(fullfile(mbd_s32k_mc_block_help('s32k14x'), 'S32K14XMCLUG.pdf'), '-browser')
      mask Display: color('black');port_label('input',1,'f16Alpha');port_label('input',2,'f16Beta');port_label('input',3,'f16ArgDcBusMsr');port_label('output',1,'f16AlphaOut');port_label('output',2,'f16BetaOut');color('black');disp('GMCLIB_ElimDcBusRip_F16');color('blue');text(tX,tY, 'BAM', 'horizontalAlignment', 'center');
  GMCLIB_ParkInv_F16 : Subsystem  mask(GMCLIB_ParkInv_F16){}
      mask help: Bit accurate model of Inverse Park transformation 2ph rotational -> 2ph stationary.
      mask init:
      | pos = get_param(gcb, 'Position');width = pos(3) - pos(1); height = pos(4) - pos(2);tX=width/2;tY=height*0.9;
      mask Help: web(fullfile(mbd_s32k_mc_block_help('s32k14x'), 'S32K14XMCLUG.pdf'), '-browser')
      mask Display: color('black');port_label('input',1,'f16D');port_label('input',2,'f16Q');port_label('input',3,'f16Sin');port_label('input',4,'f16Cos');port_label('output',1,'f16Alpha');port_label('output',2,'f16Beta');color('black');disp('GMCLIB_ParkInv_F16');color('blue');text(tX,tY, 'BAM', 'horizontalAlignment', 'center');
  GMCLIB_Park_F16 : Subsystem  mask(GMCLIB_Park_F16){}
      mask help: Bit accurate model of Park transformation 2ph stationary -> 2ph rotational.
      mask init:
      | pos = get_param(gcb, 'Position');width = pos(3) - pos(1); height = pos(4) - pos(2);tX=width/2;tY=height*0.9;
      mask Help: web(fullfile(mbd_s32k_mc_block_help('s32k14x'), 'S32K14XMCLUG.pdf'), '-browser')
      mask Display: color('black');port_label('input',1,'f16Alpha');port_label('input',2,'f16Beta');port_label('input',3,'f16Sin');port_label('input',4,'f16Cos');port_label('output',1,'f16D');port_label('output',2,'f16Q');color('black');disp('GMCLIB_Park_F16');color('blue');text(tX,tY, 'BAM', 'horizontalAlignment', 'center');
  GMCLIB_PwmIct_F16 : Subsystem  mask(GMCLIB_PwmIct_F16){}
      mask help: Bit accurate model of General Sinusoidal PWM.
      mask init:
      | pos = get_param(gcb, 'Position');width = pos(3) - pos(1); height = pos(4) - pos(2);tX=width/2;tY=height*0.9;
      mask Help: web(fullfile(mbd_s32k_mc_block_help('s32k14x'), 'S32K14XMCLUG.pdf'), '-browser')
      mask Display: color('black');port_label('input',1,'f16In1');port_label('input',2,'f16In2');port_label('output',1,'f16Out1');port_label('output',2,'f16Out2');port_label('output',3,'f16Out3');port_label('output',4,'u16Sector');color('black');disp('GMCLIB_PwmIct_F16');color('blue');text(tX,tY, 'BAM', 'horizontalAlignment', 'center');
  GMCLIB_SvmStd_F16 : Subsystem  mask(GMCLIB_SvmStd_F16){}
      mask help: Bit accurate model of Standard Space Vector Modulation.
      mask init:
      | pos = get_param(gcb, 'Position');width = pos(3) - pos(1); height = pos(4) - pos(2);tX=width/2;tY=height*0.9;
      mask Help: web(fullfile(mbd_s32k_mc_block_help('s32k14x'), 'S32K14XMCLUG.pdf'), '-browser')
      mask Display: color('black');port_label('input',1,'f16In1');port_label('input',2,'f16In2');port_label('output',1,'f16Out1');port_label('output',2,'f16Out2');port_label('output',3,'f16Out3');port_label('output',4,'u16Sector');color('black');disp('GMCLIB_SvmStd_F16');color('blue');text(tX,tY, 'BAM', 'horizontalAlignment', 'center');
  GMCLIB_SvmU0n_F16 : Subsystem  mask(GMCLIB_SvmU0n_F16){}
      mask help: Bit accurate model of Standard Space Vector Modulation.
      mask init:
      | pos = get_param(gcb, 'Position');width = pos(3) - pos(1); height = pos(4) - pos(2);tX=width/2;tY=height*0.9;
      mask Help: web(fullfile(mbd_s32k_mc_block_help('s32k14x'), 'S32K14XMCLUG.pdf'), '-browser')
      mask Display: color('black');port_label('input',1,'f16In1');port_label('input',2,'f16In2');port_label('output',1,'f16Out1');port_label('output',2,'f16Out2');port_label('output',3,'f16Out3');port_label('output',4,'u16Sector');color('black');disp('GMCLIB_SvmU0n_F16');color('blue');text(tX,tY, 'BAM', 'horizontalAlignment', 'center');
